simulink model "state_tester"  (R2019a)
settings: Solver=VariableStepAuto  StartTime=0.0  StopTime=10.0  RelTol=1e-3
values from neighbouring files (symbols this model uses):
  A1 = [(-Ra/La) ((-ka*ia)/La); ((ka*ia)/J) (-B/J)]    [ex2.m]    (also in ex3.m = [(-Ra/La) ((-ka*ia)/La); (ka*ia)/J -(B/J)])
  A_fs = [-0.5 0 -455;0 -2.9 455; 1 -1 0]    [ex4.m]    (also in ex5.m; ex5test.m)
  B1 = [(1/La) 0; 0 (-1/J)]    [ex2.m]    (also in ex3.m)
  B_fs = [17 0; 0 -5; 0 0]    [ex4.m]    (also in ex5.m; ex5test.m)
  C1 = [1 0;0 1]    [ex2.m]    (also in ex3.m)
  C_fs = [1 0 0; 0 1 0; 0 0 1]    [ex4.m]    (also in ex5.m; ex5test.m)
  D1 = [0 0;0 0]    [ex2.m]    (also in ex3.m)
  D_fs = [0 0;0 0; 0 0]    [ex4.m]    (also in ex5.m; ex5test.m)
  k = place(open_A1, open_B1, p2)    [ex2.m]
settings Model: Creator=kecy6rkk  LastModifiedBy=kecy6rkk

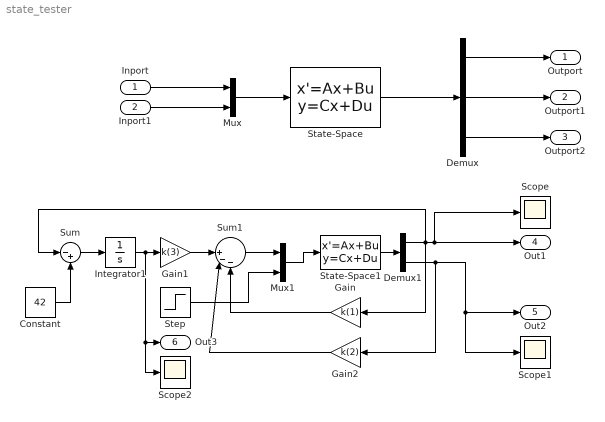
== system state_tester ==
  Inport : Inport
  Inport1 : Inport  Port=2
  Constant : Constant  Value=42
  Demux : Demux  Outputs=3
  Demux1 : Demux  Outputs=2
  Gain : Gain  Gain=k(1)
  Gain1 : Gain  Gain=k(3)
  Gain2 : Gain  Gain=k(2)
  Integrator1 : Integrator
  Mux : Mux  Inputs=2
  Mux1 : Mux  Inputs=2
  Scope : Scope
  Scope1 : Scope
  Scope2 : Scope
  State-Space : StateSpace  A=A_fs  B=B_fs  C=C_fs  D=D_fs  InitialCondition=0
  State-Space1 : StateSpace  A=A1  B=B1  C=C1  D=D1  InitialCondition=0
  Step : Step  Time=0  After=75  SampleTime=0
  Sum : Sum  Inputs=|-+
  Sum1 : Sum  Inputs=||+--
  Outport : Outport
  Outport1 : Outport  Port=2
  Outport2 : Outport  Port=3
  Out1 : Outport  Port=4
  Out2 : Outport  Port=5
  Out3 : Outport  Port=6
  wires:
  State-Space/1 -> Demux/1
  Mux/1 -> State-Space/1
  Demux/3 -> Outport2/1
  Demux/2 -> Outport1/1
  Demux/1 -> Outport/1
  Inport1/1 -> Mux/2
  Inport/1 -> Mux/1
  Step/1 -> Mux1/2
  Gain1/1 -> Sum1/1
  Sum1/1 -> Mux1/1
  Mux1/1 -> State-Space1/1
  Demux1/1 -> Sum/1, Gain/1, Scope/1, Out1/1
  Gain/1 -> Sum1/3
  Gain2/1 -> Sum1/2
  State-Space1/1 -> Demux1/1
  Demux1/2 -> Gain2/1, Out2/1, Scope1/1
  Integrator1/1 -> Scope2/1, Out3/1, Gain1/1
  Constant/1 -> Sum/2
  Sum/1 -> Integrator1/1
